simulink model "gm_ADC_RAW_TO_VALUE"  (R2018a)
settings: Solver=FixedStepDiscrete  StartTime=0.0  StopTime=SimulationsDauer  RelTol=1e-3  EnableMultiTasking=on
undefined symbols (not defined in the file or in its folder): ADC_SET_USER_OFFSET, ADC_USER_OFFSET, T_mech
settings Model: Creator=zedboard  LastModifiedBy=Wendel
settings OptimizationCC: BlockReduction=off  ConditionallyExecuteInputs=off  DefaultParameterBehavior=Inlined  LifeSpan=inf
settings DebuggingCC: AlgebraicLoopMsg=error  InheritedTsInSrcMsg=none  SFUnexpectedBacktrackingDiag=warning  SFNoUnconditionalDefaultTransitionDiag=warning  SFExecutionAtInitializationDiag=none
settings HardwareCC: ProdBitPerPointer=32  ProdBitPerSizeT=32  ProdBitPerPtrDiffT=32  ProdLargestAtomicFloat=None  ProdIntDivRoundTo=Undefined  ProdEndianess=Unspecified  ProdWordSize=32  ProdHWDeviceType=ASIC/FPGA->ASIC/FPGA  ProdEqTarget=off
settings CodeAppCC: StateflowObjectComments=on
settings GRTTargetCC: TargetLangStandard=C89/C90 (ANSI)  GeneratePreprocessorConditionals=Disable all
settings ConfigComp: CovMetricSettings=dw  CovHtmlReporting=on  CovSaveCumulativeToWorkspaceVar=on  CovSaveSingleToWorkspaceVar=on  CovExternalEMLEnable=off

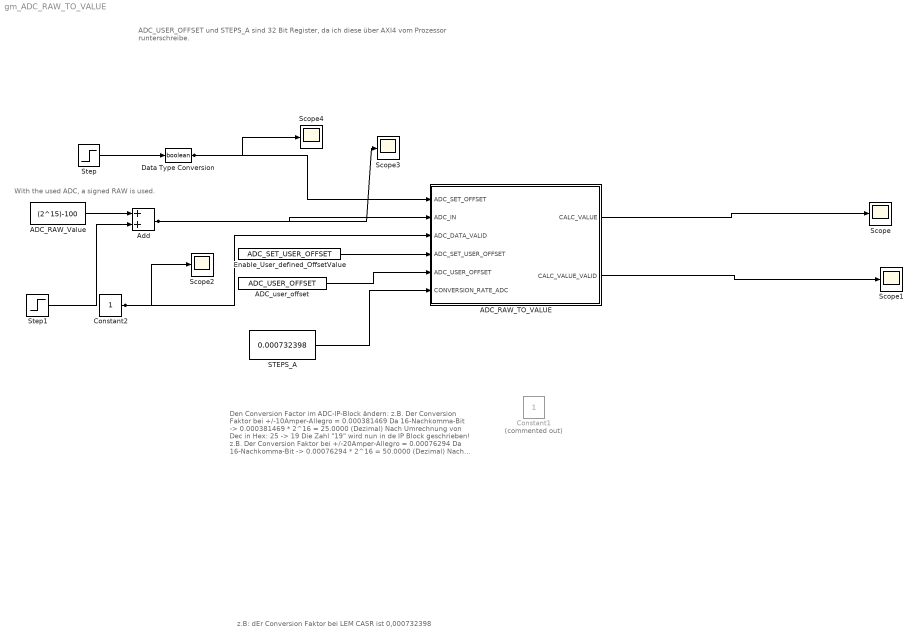
== system gm_ADC_RAW_TO_VALUE ==
  note: Den Conversion Factor im ADC-IP-Block ändern:
      |
      | z.B. Der Conversion Faktor bei +/-10Amper-Allegro = 0.000381469
      | Da 16-Nachkomma-Bit -> 0.000381469 * 2^16 = 25.0000 (Dezimal)
      | Nach Umrechnung von Dec in Hex: 25 -> 19
      | Die Zahl "19" wird nun in de IP Block geschrieben!
      |
      | z.B. Der Conversion Faktor bei +/-20Amper-Allegro = 0.00076294
      | Da 16-Nachkomma-Bit -> 0.00076294 * 2^16 = 50.0000 (Dezimal)
      | Nach Umrechnung von Dec in Hex: 50 -> 32
      | Die Zahl "32" wird nun in de IP Block geschrieben!
      |
      |
      | z.B. Der Conversion Faktor bei Chile Stromsensor = 0.00041018
      | Da 16-Nachkomma-Bit -> 0.00041018 * 2^16 = 26.8816 (Dezimal)
      | Nach Umrechnung von Dec in Hex:  27 -> 1B
      | Die Zahl "1B" wird nun in de IP Block geschrieben!
  note: z.B: dEr Conversion Faktor bei LEM CASR ist 0,000732398
  note: With the used ADC, a signed RAW is used.
  note: ADC_USER_OFFSET und STEPS_A sind 32 Bit Register, da ich diese über AXI4 vom Prozessor runterschreibe.
  ADC_RAW_TO_VALUE : Subsystem
  ADC_RAW_Value : Constant  Value=(2^15)-100  OutDataTypeStr=fixdt(1,16,0)  SampleTime=T_mech
  ADC_user_offset : Constant  Value=ADC_USER_OFFSET  OutDataTypeStr=fixdt(1,32,0)  SampleTime=-1
  Add : Sum  OutDataTypeStr=Inherit: Same as first input
  Constant1 : Constant  Commented=on  OutDataTypeStr=boolean
  Constant2 : Constant  OutDataTypeStr=boolean  SampleTime=T_mech
  Data Type Conversion : DataTypeConversion  OutDataTypeStr=boolean
  Enable_User_defined_OffsetValue : Constant  Value=ADC_SET_USER_OFFSET  OutDataTypeStr=boolean  SampleTime=T_mech
  STEPS_A : Constant  Value=0.000732398  OutDataTypeStr=fixdt(1,32,32)  SampleTime=-1
  Scope{,1..4} (5 alike) : Scope
  Step : Step  Time=0.01  Before=1  After=0  SampleTime=T_mech
  Step1 : Step  Time=0.02  After=50  SampleTime=T_mech
  wires:
  STEPS_A/1 -> ADC_RAW_TO_VALUE/6(CONVERSION_RATE_ADC)
  ADC_user_offset/1 -> ADC_RAW_TO_VALUE/5(ADC_USER_OFFSET)
  Enable_User_defined_OffsetValue/1 -> ADC_RAW_TO_VALUE/4(ADC_SET_USER_OFFSET)
  Data Type Conversion/1 -> ADC_RAW_TO_VALUE/1(ADC_SET_OFFSET), Scope4/1
  Step1/1 -> Add/2
  ADC_RAW_Value/1 -> Add/1
  ADC_RAW_TO_VALUE/2(CALC_VALUE_VALID) -> Scope1/1
  Constant2/1 -> ADC_RAW_TO_VALUE/3(ADC_DATA_VALID), Scope2/1
  Add/1 -> ADC_RAW_TO_VALUE/2(ADC_IN), Scope3/1
  Step/1 -> Data Type Conversion/1
  ADC_RAW_TO_VALUE/1(CALC_VALUE) -> Scope/1

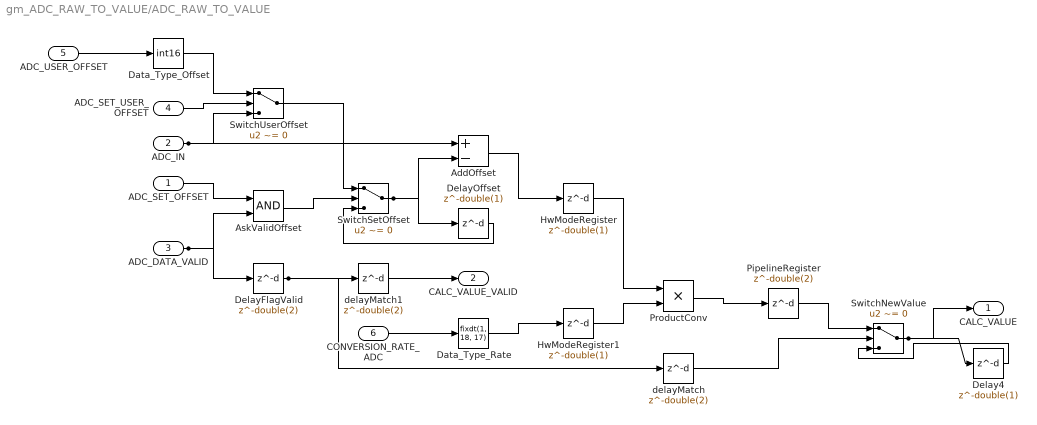
== system gm_ADC_RAW_TO_VALUE/ADC_RAW_TO_VALUE ==
  ADC_SET_OFFSET : Inport  OutDataTypeStr=boolean  PortDimensions=1  SampleTime=1e-07
  ADC_IN : Inport  Port=2  OutDataTypeStr=int16  PortDimensions=1  SampleTime=1e-07
  ADC_DATA_VALID : Inport  Port=3  OutDataTypeStr=boolean  PortDimensions=1  SampleTime=1e-07
  ADC_SET_USER_OFFSET : Inport  Port=4  OutDataTypeStr=boolean  PortDimensions=1  SampleTime=1e-07
  ADC_USER_OFFSET : Inport  Port=5  OutDataTypeStr=int32  PortDimensions=1  SampleTime=1e-07
  CONVERSION_RATE_ADC : Inport  Port=6  OutDataTypeStr=fixdt(1, 32, 32)  PortDimensions=1  SampleTime=1e-07
  AddOffset : Sum  Inputs=+-  AccumDataTypeStr=fixdt(1, 18, 0)  OutDataTypeStr=fixdt(1, 18, 0)  SampleTime=1e-07
  AskValidOffset : Logic  AllPortsSameDT=off  OutDataTypeStr=boolean  SampleTime=1e-07
  Data_Type_Offset : DataTypeConversion  OutDataTypeStr=int16  SampleTime=1e-07
  Data_Type_Rate : DataTypeConversion  OutDataTypeStr=fixdt(1, 18, 17)  SampleTime=1e-07
  Delay4 : Delay  DelayLength=double(1)  InitialCondition=0  InputProcessing=Inherited  SampleTime=1e-07
  DelayFlagValid : Delay  DelayLength=double(2)  InitialCondition=0  InputProcessing=Inherited  SampleTime=1e-07
  DelayOffset : Delay  DelayLength=double(1)  InitialCondition=0  InputProcessing=Inherited  SampleTime=1e-07
  HwModeRegister : Delay  DelayLength=double(1)  InitialCondition=0  InputProcessing=Inherited  SampleTime=1e-07
  HwModeRegister1 : Delay  DelayLength=double(1)  InitialCondition=0  InputProcessing=Inherited  SampleTime=1e-07
  PipelineRegister : Delay  DelayLength=double(2)  InitialCondition=0  InputProcessing=Inherited  SampleTime=1e-07
  ProductConv : Product  Inputs=**  OutDataTypeStr=fixdt(1, 18, 11)  SampleTime=1e-07
  SwitchNewValue : Switch  Criteria=u2 ~= 0  Threshold=double(0)  OutDataTypeStr=fixdt(1, 18, 11)  SampleTime=1e-07
  SwitchSetOffset : Switch  Criteria=u2 ~= 0  Threshold=double(0)  OutDataTypeStr=int16  SampleTime=1e-07
  SwitchUserOffset : Switch  Criteria=u2 ~= 0  Threshold=double(0)  OutDataTypeStr=int16  SampleTime=1e-07
  delayMatch : Delay  DelayLength=double(2)  InitialCondition=0  InputProcessing=Inherited  SampleTime=1e-07
  delayMatch1 : Delay  DelayLength=double(2)  InitialCondition=0  InputProcessing=Inherited  SampleTime=1e-07
  CALC_VALUE : Outport
  CALC_VALUE_VALID : Outport  Port=2
  wires:
  ADC_SET_OFFSET/1 -> AskValidOffset/1
  ADC_IN/1 -> SwitchUserOffset/3, AddOffset/1
  ADC_DATA_VALID/1 -> AskValidOffset/2, DelayFlagValid/1
  ADC_SET_USER_OFFSET/1 -> SwitchUserOffset/2
  ADC_USER_OFFSET/1 -> Data_Type_Offset/1
  CONVERSION_RATE_ADC/1 -> Data_Type_Rate/1
  AddOffset/1 -> HwModeRegister/1
  AskValidOffset/1 -> SwitchSetOffset/2
  Data_Type_Offset/1 -> SwitchUserOffset/1
  Data_Type_Rate/1 -> HwModeRegister1/1
  delayMatch/1 -> SwitchNewValue/2
  PipelineRegister/1 -> SwitchNewValue/1
  SwitchSetOffset/1 -> AddOffset/2, DelayOffset/1
  SwitchUserOffset/1 -> SwitchSetOffset/1
  delayMatch1/1 -> CALC_VALUE_VALID/1
  DelayFlagValid/1 -> delayMatch1/1, delayMatch/1
  DelayOffset/1 -> SwitchSetOffset/3
  Delay4/1 -> SwitchNewValue/3
  SwitchNewValue/1 -> Delay4/1, CALC_VALUE/1
  ProductConv/1 -> PipelineRegister/1
  HwModeRegister/1 -> ProductConv/1
  HwModeRegister1/1 -> ProductConv/2
